simulink model "Wall_Model_Version_Final_2018a"  (R2018a)
settings: Solver=ode3  StartTime=0.0  StopTime=87000  FixedStep=Ts  RelTol=1e-3  EnableMultiTasking=on
InitFcn:
  | clc;
  | clear all;
  | close all;
  | addpath('D:\Aravind_A0164966M_EE5003\Matlab files\3r2c model')
  | Ts=1
  | Duration=36000;
  | %% Coefficients of Rs and Cs
  | 
  | %% Front Wall
  | l1 = 7.37;
  | b1 = 2.63;
  | y1 = 0.186;
  | x1 = 0.111;
  | y2 = 0.814;
  | x2 = 0.506;
  | x3 = 0.383;
  | 
  | %% Left Wall
  | l2 = 10.11;
  | b2 = 2.63;
  | y3 = 0.186;
  | x4 = 0.111;
  | y4 = 0.814;
  | x5 = 0.506;
  | x6 = 0.383;
  | 
  | %% Left Wall Glass
  | x4_g = 0.5;
  | x5_g = 0.5;
  | y3_g = 1;
  | 
  | %% Right Wall
  | l3 = 7.37;
  | b3 = 2.63;
  | y5 = 0.186;
  | x7 = 0.111;
  | y6 = 0.814;
  | x8 = 0.506;
  | x9 = 0.383;
  | 
  | %% Back Wall
  | l4 = 10.11;
  | b4 = 2.63;
  | y7 = 1;
  | x10 = 0.5;
  | %y8 = 0.5;
  | x11 = 0.5;
  | %x12= 0.33;
  | 
  | %% Roof
  | l5 = 10.11;
  | b5 = 7.37;
  | y9 = 0.186;
  | x13 = 0.111;
  | y10 = 0.814;
  | x14 = 0.506;
  | x15 = 0.383;
  | 
  | %% Floor
  | l6 = 10.11;
  | b6 = 7.37;
  | y11 = 0.186;
  | x16 = 0.111;
  | y12 = 0.814;
  | x17 = 0.506;
  | x18 = 0.383;
  | 
  | %%Areas
  | A1 = l1 * b1;
  | A2 = l2 * b2;
  | A3 = l3 * b3;
  | A4 = l4 * b4;
  | A5 = l5 * b5;
  | A6 = l6 * b6;
  | 
  | %% Initial Temperatures at the surfaces
  | T1_initial_front=301;
  | T2_initial_front=300;
  | 
  | T1_initial_left=301;
  | T2_initial_left=300;
  | 
  | T1_initial_right=301;
  | T2_initial_right=300;
  | 
  | T1_initial_back=301;
  | T2_initial_back=300;
  | 
  | T1_initial_roof=301;
  | T2_initial_roof=300;
  | 
  | T1_initial_floor=301;
  | T2_initial_floor=300;
  | 
  | %ri = 0.1300; % m2 K/W resistance of inner surface of brick wall
  | %rso = 0.04; % m2 K/W resistance of outer surface of the wall
  | 
  | ri = 0;
  | rso = 0;
  | %% Density of Building materials in the room
  | p_conc    = 2400; % kg/m3 density of concrete
  | p_pstr     = 850; % kg/m3 density of plastering
  | p_gb       = 1100; % kg/m3 density of gypsum board
  | p_glass    = 2530; % kg/m3 density of glass
  | p_swood  = 550;   % kg/m3 density of soft-wood
  | 
  | %% Thermal heat capacity of the building materials in the room
  | c_conc    = 840;  % J/kg K heat capacity of concrete
  | c_pstr     = 1000;  %J/kg K heat capacity of plastering
  | c_gb       = 700; % J/kg K heat capacity of gypsum board
  | c_glass    = 840;  % J/kg K heat capacity of glass
  | c_swood  = 1700; % J/kg K heat capacity of soft-wood
  | 
  | %% Thermal conductivity(lamda) of building materials in the room
  | l_conc    = 0.8;  % W/m K Thermal conductivity of concrete
  | l_pstr     = 0.013;  % W/m K Thermal conductivity of plastering
  | l_gb       = 0.35; % W/m K Thermal conductivity of gypsum board
  | l_glass    = 0.8;  % W/m K Thermal conductivity of glass
  | l_swood  = 0.08; % W/m K Thermal conductivity of soft-wood
  | 
  | %% Standard thickness of materials used
  | d_conc = 0.01;  % m Thickness of concrete BCA standard
  | d_pstr = 0.005; % m Thickness of plastering BCA standard
  | d_glass = 0.015; % m Thickness of glass wall widely used
  | d_swood = 0.01; % m Thickness of softwood on the right wall
  | d_gb = 0.015; % m Thickness of gypsum board
  | 
  | %% Resistance and Capacitance of front Wall
  | Rth1 =( ri + rso + (d_conc/l_conc) + (d_pstr/l_pstr))/(A1); % Thermal resistance
  | Cth1 = A1*(d_conc*p_conc*c_conc + d_pstr*p_pstr*c_pstr) ; % Thermal Capacitance
  | 
  | %% Resistance and Capacitance of left Wall concrete
  | A_conc = A2 * 0.5; % Half of the wall on the left is  glass wall
  | Rth2 =( ri + rso + (d_conc/l_conc) + (d_pstr/l_pstr))/(A_conc); % Thermal resistance
  | Cth2 = A_conc*(d_conc*p_conc*c_conc + d_pstr*p_pstr*c_pstr); % Thermal Capacitance
  | 
  | %% Resistance and Capacitance of left Wall glass
  | A_glass = A2 * 0.5; % Half of the wall on the left is  glass wall
  | Rth2_g =(d_glass/l_glass) /(A_glass); % Thermal resistance
  | Cth2_g = A_glass*(d_glass*p_glass*c_glass ); % Thermal Capacitance
  | 
  | %% Resistance and Capacitance of right Wall
  | Rth3 = ( ri + rso+ (d_conc/l_conc) + (d_swood/l_swood))/(A3);% Thermal resistance
  | Cth3 = A3*(d_swood*p_swood*c_swood + d_conc*p_conc*c_conc ); % Thermal Capacitance
  | 
  | %% Resistance and Capacitance of back Wall
  | Rth4 =(d_glass/l_glass) /(A4); % Thermal resistance
  | Cth4 = A4*(d_glass*p_glass*c_glass ); % Thermal Capacitance
  | 
  | %% Resistance and Capacitance of roof Wall
  | Rth5 = (d_gb/l_gb)/(A5);% Thermal resistance
  | Cth5 = A5*(d_gb*p_gb*c_gb ); % Thermal Capacitance
  | 
  | %% Resistance and Capacitance of floor Wall
  | Rth6 = (d_gb/l_gb)/(A6);% Thermal resistance
  | Cth6 = A6*(d_gb*p_gb*c_gb ); % Thermal Capacitance
  | 
  | %% Volume and mass of room
  | density_of_air = 1.184; % kg/m3 at 25 deg. K
  | volume = l1*l2*b1; % m3
  | mass = volume * density_of_air ;% kg
  | specific_heat = 1.005; % J/kg deg.K
  | tic;
  | 
  | Tleft = 298;
libraries: powerlib x72, simulink x1
(part 1 of 2)
settings Model: EnablePacing=on  Creator=elekkr  LastModifiedBy=accma
settings DataIOCC: LimitDataPoints=on  SaveFormat=Array
settings OptimizationCC: LifeSpan=inf
settings DebuggingCC: UnconnectedInputMsg=none  UnconnectedOutputMsg=none  UnconnectedLineMsg=none  SFUnexpectedBacktrackingDiag=warning  SFNoUnconditionalDefaultTransitionDiag=warning  SFExecutionAtInitializationDiag=none
settings HardwareCC: ProdBitPerPointer=32  ProdBitPerSizeT=32  ProdBitPerPtrDiffT=32  ProdLargestAtomicFloat=None  ProdIntDivRoundTo=Undefined  ProdEndianess=Unspecified  ProdWordSize=32  ProdHWDeviceType=32-bit Generic
settings ModelReferenceCC: PropagateSignalLabelsOutOfModel=off
settings CodeAppCC: StateflowObjectComments=on
settings GRTTargetCC: TargetLangStandard=C89/C90 (ANSI)  GeneratePreprocessorConditionals=Disable all
settings ConfigComp: CovMetricSettings=dw  CovHtmlReporting=on  CovSaveCumulativeToWorkspaceVar=on  CovSaveSingleToWorkspaceVar=on  CovExternalEMLEnable=off
settings SimscapeCC: SimscapeNormalizeSystem=off

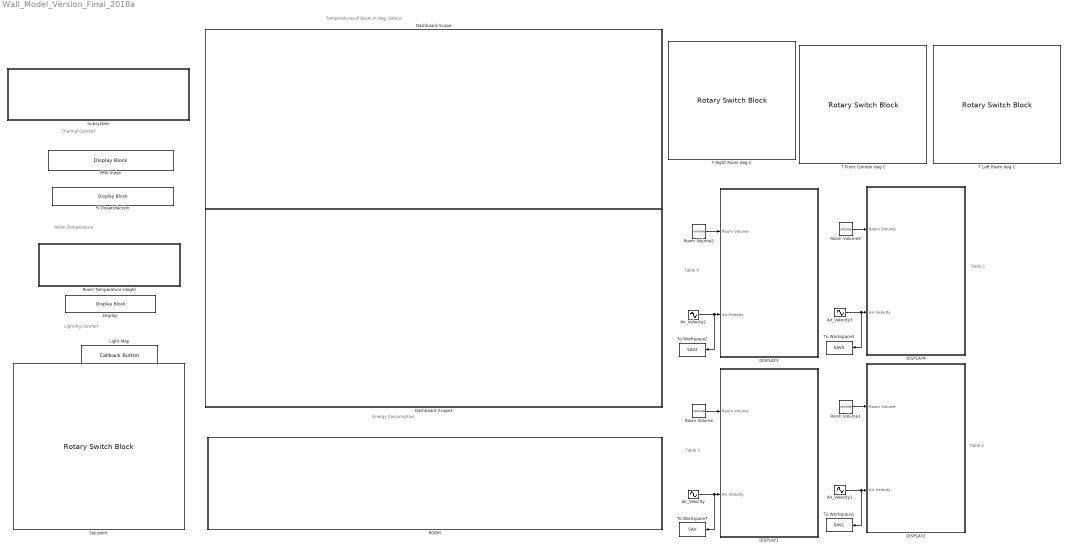
== system Wall_Model_Version_Final_2018a ==
  note: Table 1
  note: Thermal Comfort
  note: Lighting Comfort
  note: Temperatures of Room in deg. Celsius
  note: Energy Consumption
  note: Table 2
  note: Table 3
  note: Table 4
  note: Room Temperature
  % Dissatisfaction : DisplayBlock  WebBlockId=889  LabelPosition=Hide
  Air_Velocity{,1..3} (4 alike) : Sin  Amplitude=0.2  Bias=0.8  Frequency=2*pi/(12*3600)  SampleTime=0
  DISPLAY1 : Subsystem  mask(Sensor_node){}
      mask Display: fprintf('CO2 488.60 ppm\n\nCO 0.10 ppm\n\nHCHO 0.00 ppm\n\nO3 0.09 ppm\n\nPM2_5 0.03 ppm\n\nPM10 0.06 ppm\n\nAir Quality Index 14.82\n\n')
  DISPLAY2 : Subsystem  mask(Sensor_node){}
      mask Display: fprintf('CO2 491.84 ppm\n\nCO 0.11 ppm\n\nHCHO 0.00 ppm\n\nO3 0.08 ppm\n\nPM2_5 0.02 ppm\n\nPM10 0.02 ppm\n\nAir Quality Index 15.36\n\n')
  DISPLAY3 : Subsystem  mask(Sensor_node){}
      mask Display: fprintf('CO2 489.68 ppm\n\nCO 0.11 ppm\n\nHCHO 0.00 ppm\n\nO3 0.05 ppm\n\nPM2_5 0.05 ppm\n\nPM10 0.05 ppm\n\nAir Quality Index 15.00\n\n')
  DISPLAY4 : Subsystem  mask(Sensor_node){}
      mask Display: fprintf('CO2 489.68 ppm\n\nCO 0.09 ppm\n\nHCHO 0.00 ppm\n\nO3 0.08 ppm\n\nPM2_5 0.05 ppm\n\nPM10 0.04 ppm\n\nAir Quality Index 15.00\n\n')
  Dashboard Scope : Subsystem  DialogController=hmiCreateDDGDialog  IsWebBlock=on  mask(MWDashboardBlock){webBlockId=52df8120-a1fd-461c-886b-445e676d82b8, webBlockType=sdiscope, ShowInLibBrowser=on, ShowInitialText=on, HMISrcModelName=Wall_Model_Version_Final_2018a}
      mask prompts: webBlockId "WebBlock Id"; webBlockType "WebBlock Type"; HMISrcModelName "Source Model"
      mask help: Traces signals on the dashboard scope during simulation.
      mask Help: helpview([docroot '/mapfiles/simulink.map'], 'hmi_scope')
      mask Display:
      | if strcmp(get_param(bdroot(gcb),'BlockDiagramType'),'library')
      |  image([(matlabroot) '/toolbox/simulink/hmi/icons/SDIScope.png'])
      | end
  Dashboard Scope1 : Subsystem  DialogController=hmiCreateDDGDialog  IsWebBlock=on  mask(MWDashboardBlock){webBlockId=c0c79143-6636-452e-a0ed-83ee40a087d1, webBlockType=sdiscope, ShowInLibBrowser=on, ShowInitialText=on, HMISrcModelName=Wall_Model_Version_Final_2018a}
      mask prompts: webBlockId "WebBlock Id"; webBlockType "WebBlock Type"; HMISrcModelName "Source Model"
      mask help: Traces signals on the dashboard scope during simulation.
      mask Help: helpview([docroot '/mapfiles/simulink.map'], 'hmi_scope')
      mask Display:
      | if strcmp(get_param(bdroot(gcb),'BlockDiagramType'),'library')
      |  image([(matlabroot) '/toolbox/simulink/hmi/icons/SDIScope.png'])
      | end
  Display : DisplayBlock  WebBlockId=772  LabelPosition=Hide
  Light Map : CallbackButton  WebBlockId=904
      settings: ClickFcn=heatmap_V2
  PMV Index : DisplayBlock  WebBlockId=888  LabelPosition=Hide
  ROOM : Subsystem
  Room Temperature (degK) : Subsystem  DialogController=hmiCreateDDGDialog  IsWebBlock=on  mask(MWDashboardBlock){webBlockId=d421009d-199f-4938-a325-427fcb2645d5, webBlockType=lineargauge, ShowInLibBrowser=on, ShowInitialText=on, HMISrcModelName=Wall_Model_Version_Final_2018a}
      mask prompts: webBlockId "WebBlock Id"; webBlockType "WebBlock Type"; HMISrcModelName "Source Model"
      mask help: Display an input value on a linear scale.
      mask Help: helpview([docroot '/mapfiles/simulink.map'], 'hmi_linear_gauge')
      mask Display:
      | if strcmp(get_param(bdroot(gcb),'BlockDiagramType'),'library')
      |  image([(matlabroot) '/toolbox/simulink/hmi/icons/LinearGauge.png'])
      | end
  Room Volume{,1..3} (4 alike) : Constant  Value=volume
  Set-point : RotarySwitchBlock  WebBlockId=542  LabelPosition=Hide
      settings: Values={{'Cold', '', '', 'Optimum', '', '', '', '', '', '', 'Hot'}, [293 294 295 296 297 298 299 300 301 302 303]}
  Subsystem : Subsystem  mask(GBIC_Simulation time){}
      settings: AttributesFormatString=58.23
      mask Display: fprintf('Simulation_Time_Elapsed=28.00 seconds\nPhysical_Time_Elapsed=58.23 seconds\nSimulation_Speed=0.48 times')
  T Front Corridor deg.C : RotarySwitchBlock  WebBlockId=766  LabelPosition=Hide
      settings: Values={{'20', '21', '22', '23', '24', '25', '26', '27', '28', '29', '30', '31', '32'}, [293 294 295 296 297 298 299 300 301 302 303 304 305]}
  T Left Room deg.C : RotarySwitchBlock  WebBlockId=768  LabelPosition=Hide
      settings: Values={{'20', '21', '22', '23', '24', '25', '26', '27', '28', '29', '30', '31', '32'}, [293 294 295 296 297 298 299 300 301 302 303 304 305]}
  T Right Room deg.C : RotarySwitchBlock  WebBlockId=769  LabelPosition=Hide
      settings: Values={{'20', '21', '22', '23', '24', '25', '26', '27', '28', '29', '30', '31', '32'}, [293 294 295 296 297 298 299 300 301 302 303 304 305]}
  To Workspace1 : ToWorkspace  VariableName=SAV1  SaveFormat=Timeseries  SampleTime=-1
  To Workspace2 : ToWorkspace  VariableName=SAV2  SaveFormat=Timeseries  SampleTime=-1
  To Workspace3 : ToWorkspace  VariableName=SAV3  SaveFormat=Timeseries  SampleTime=-1
  To Workspace7 : ToWorkspace  VariableName=SAV  SaveFormat=Timeseries  SampleTime=-1
  wires:
  Room Volume/1 -> DISPLAY1/1(Room Volume)
  Air_Velocity/1 -> To Workspace7/1, DISPLAY1/2(Air Velocity)
  Air_Velocity1/1 -> To Workspace1/1, DISPLAY2/2(Air Velocity)
  Room Volume1/1 -> DISPLAY2/1(Room Volume)
  Air_Velocity2/1 -> To Workspace2/1, DISPLAY3/2(Air Velocity)
  Room Volume2/1 -> DISPLAY3/1(Room Volume)
  Room Volume3/1 -> DISPLAY4/1(Room Volume)
  Air_Velocity3/1 -> To Workspace3/1, DISPLAY4/2(Air Velocity)

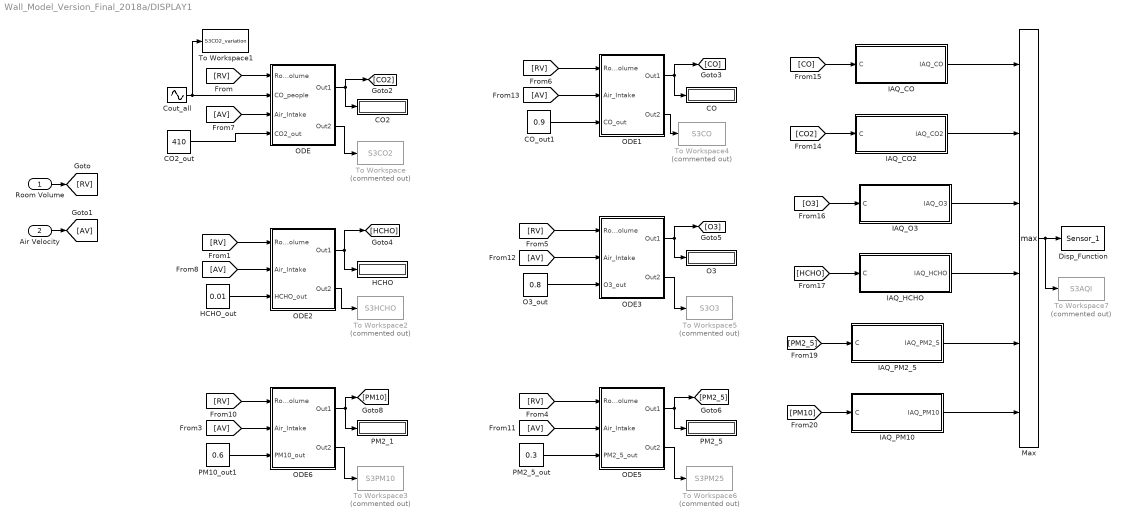
== system Wall_Model_Version_Final_2018a/DISPLAY1 ==
  Room Volume : Inport
  Air Velocity : Inport  Port=2
  CO : Display
  CO2 : Display
  CO2_out : Constant  Value=410
  CO_out1 : Constant  Value=0.9
  Cout_all : Sin  Amplitude=50  Bias=450  Frequency=2*pi/(24*3600)  SampleTime=0
  Disp_Function : M-S-Function  FunctionName=Sensor_1
  HCHO : Display
  HCHO_out : Constant  Value=0.01
  IAQ_CO : MATLAB Function  TreatAsAtomicUnit=on
  IAQ_CO2 : MATLAB Function  TreatAsAtomicUnit=on
  IAQ_HCHO : MATLAB Function  TreatAsAtomicUnit=on
  IAQ_O3 : MATLAB Function  TreatAsAtomicUnit=on
  IAQ_PM10 : MATLAB Function  TreatAsAtomicUnit=on
  IAQ_PM2_5 : MATLAB Function  TreatAsAtomicUnit=on
  Max : MinMax  Function=max  Inputs=6
  O3 : Display
  O3_out : Constant  Value=0.8
  ODE : Subsystem
  ODE1 : Subsystem
  ODE2 : Subsystem
  ODE3 : Subsystem
  ODE5 : Subsystem
  ODE6 : Subsystem
  PM10_out1 : Constant  Value=0.6
  PM2_1 : Display
  PM2_5 : Display
  PM2_5_out : Constant  Value=0.3
  To Workspace : ToWorkspace  Commented=on  VariableName=S3CO2  SaveFormat=Timeseries  SampleTime=-1
  To Workspace1 : ToWorkspace  VariableName=S3CO2_variation  SaveFormat=Timeseries  SampleTime=-1
  To Workspace2 : ToWorkspace  Commented=on  VariableName=S3HCHO  SaveFormat=Timeseries  SampleTime=-1
  To Workspace3 : ToWorkspace  Commented=on  VariableName=S3PM10  SaveFormat=Timeseries  SampleTime=-1
  To Workspace4 : ToWorkspace  Commented=on  VariableName=S3CO  SaveFormat=Timeseries  SampleTime=-1
  To Workspace5 : ToWorkspace  Commented=on  VariableName=S3O3  SaveFormat=Timeseries  SampleTime=-1
  To Workspace6 : ToWorkspace  Commented=on  VariableName=S3PM25  SaveFormat=Timeseries  SampleTime=-1
  To Workspace7 : ToWorkspace  Commented=on  VariableName=S3AQI  SaveFormat=Timeseries  SampleTime=-1
  wires:
  Cout_all/1 -> To Workspace1/1, ODE/2(CO_people)
  ODE2/1(Out1) -> HCHO/1, [HCHO]
  HCHO_out/1 -> ODE2/3(HCHO_out)
  CO_out1/1 -> ODE1/3(CO_out)
  CO2_out/1 -> ODE/4(CO2_out)
  O3_out/1 -> ODE3/3(O3_out)
  ODE3/1(Out1) -> O3/1, [O3]
  IAQ_CO/1(IAQ_CO) -> Max/1
  IAQ_HCHO/1(IAQ_HCHO) -> Max/4
  ODE/1(Out1) -> CO2/1, [CO2]
  IAQ_CO2/1(IAQ_CO2) -> Max/2
  ODE1/1(Out1) -> CO/1, [CO]
  IAQ_O3/1(IAQ_O3) -> Max/3
  ODE5/1(Out1) -> PM2_5/1, [PM2_5]
  PM2_5_out/1 -> ODE5/3(PM2_5_out)
  [RV] -> ODE/1(Room_Volume)
  [RV] -> ODE2/1(Room_Volume)
  [RV] -> ODE5/1(Room_Volume)
  [RV] -> ODE3/1(Room_Volume)
  [RV] -> ODE1/1(Room_Volume)
  [AV] -> ODE/3(Air_Intake)
  [AV] -> ODE2/2(Air_Intake)
  [AV] -> ODE5/2(Air_Intake)
  [AV] -> ODE3/2(Air_Intake)
  [AV] -> ODE1/2(Air_Intake)
  [AV] -> ODE6/2(Air_Intake)
  [RV] -> ODE6/1(Room_Volume)
  PM10_out1/1 -> ODE6/3(PM10_out)
  [CO2] -> IAQ_CO2/1(C)
  [CO] -> IAQ_CO/1(C)
  [O3] -> IAQ_O3/1(C)
  [HCHO] -> IAQ_HCHO/1(C)
  [PM2_5] -> IAQ_PM2_5/1(C)
  [PM10] -> IAQ_PM10/1(C)
  ODE6/1(Out1) -> PM2_1/1, [PM10]
  Max/1 -> To Workspace7/1, Disp_Function/1
  IAQ_PM2_5/1(IAQ_PM2_5) -> Max/5
  IAQ_PM10/1(IAQ_PM10) -> Max/6
  Room Volume/1 -> [RV]
  Air Velocity/1 -> [AV]
  ODE/2(Out2) -> To Workspace/1
  ODE2/2(Out2) -> To Workspace2/1
  ODE6/2(Out2) -> To Workspace3/1
  ODE1/2(Out2) -> To Workspace4/1
  ODE3/2(Out2) -> To Workspace5/1
  ODE5/2(Out2) -> To Workspace6/1

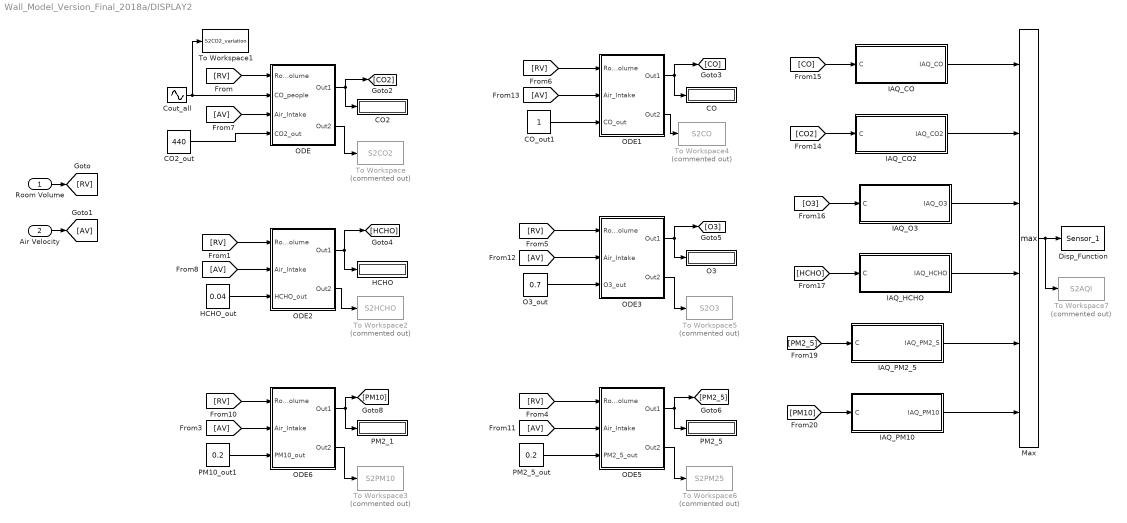
== system Wall_Model_Version_Final_2018a/DISPLAY2 ==
  Room Volume : Inport
  Air Velocity : Inport  Port=2
  CO : Display
  CO2 : Display
  CO2_out : Constant  Value=440
  CO_out1 : Constant
  Cout_all : Sin  Amplitude=50  Bias=450  Frequency=2*pi/(24*3600)  SampleTime=0
  Disp_Function : M-S-Function  FunctionName=Sensor_1
  HCHO : Display
  HCHO_out : Constant  Value=0.04
  IAQ_CO : MATLAB Function  TreatAsAtomicUnit=on
  IAQ_CO2 : MATLAB Function  TreatAsAtomicUnit=on
  IAQ_HCHO : MATLAB Function  TreatAsAtomicUnit=on
  IAQ_O3 : MATLAB Function  TreatAsAtomicUnit=on
  IAQ_PM10 : MATLAB Function  TreatAsAtomicUnit=on
  IAQ_PM2_5 : MATLAB Function  TreatAsAtomicUnit=on
  Max : MinMax  Function=max  Inputs=6
  O3 : Display
  O3_out : Constant  Value=0.7
  ODE : Subsystem
  ODE1 : Subsystem
  ODE2 : Subsystem
  ODE3 : Subsystem
  ODE5 : Subsystem
  ODE6 : Subsystem
  PM10_out1 : Constant  Value=0.2
  PM2_1 : Display
  PM2_5 : Display
  PM2_5_out : Constant  Value=0.2
  To Workspace : ToWorkspace  Commented=on  VariableName=S2CO2  SaveFormat=Timeseries  SampleTime=-1
  To Workspace1 : ToWorkspace  VariableName=S2CO2_variation  SaveFormat=Timeseries  SampleTime=-1
  To Workspace2 : ToWorkspace  Commented=on  VariableName=S2HCHO  SaveFormat=Timeseries  SampleTime=-1
  To Workspace3 : ToWorkspace  Commented=on  VariableName=S2PM10  SaveFormat=Timeseries  SampleTime=-1
  To Workspace4 : ToWorkspace  Commented=on  VariableName=S2CO  SaveFormat=Timeseries  SampleTime=-1
  To Workspace5 : ToWorkspace  Commented=on  VariableName=S2O3  SaveFormat=Timeseries  SampleTime=-1
  To Workspace6 : ToWorkspace  Commented=on  VariableName=S2PM25  SaveFormat=Timeseries  SampleTime=-1
  To Workspace7 : ToWorkspace  Commented=on  VariableName=S2AQI  SaveFormat=Timeseries  SampleTime=-1
  wires:
  Cout_all/1 -> To Workspace1/1, ODE/2(CO_people)
  ODE2/1(Out1) -> HCHO/1, [HCHO]
  HCHO_out/1 -> ODE2/3(HCHO_out)
  CO_out1/1 -> ODE1/3(CO_out)
  CO2_out/1 -> ODE/4(CO2_out)
  O3_out/1 -> ODE3/3(O3_out)
  ODE3/1(Out1) -> O3/1, [O3]
  IAQ_CO/1(IAQ_CO) -> Max/1
  IAQ_HCHO/1(IAQ_HCHO) -> Max/4
  ODE/1(Out1) -> CO2/1, [CO2]
  IAQ_CO2/1(IAQ_CO2) -> Max/2
  ODE1/1(Out1) -> CO/1, [CO]
  IAQ_O3/1(IAQ_O3) -> Max/3
  ODE5/1(Out1) -> PM2_5/1, [PM2_5]
  PM2_5_out/1 -> ODE5/3(PM2_5_out)
  [RV] -> ODE/1(Room_Volume)
  [RV] -> ODE2/1(Room_Volume)
  [RV] -> ODE5/1(Room_Volume)
  [RV] -> ODE3/1(Room_Volume)
  [RV] -> ODE1/1(Room_Volume)
  [AV] -> ODE/3(Air_Intake)
  [AV] -> ODE2/2(Air_Intake)
  [AV] -> ODE5/2(Air_Intake)
  [AV] -> ODE3/2(Air_Intake)
  [AV] -> ODE1/2(Air_Intake)
  [AV] -> ODE6/2(Air_Intake)
  [RV] -> ODE6/1(Room_Volume)
  PM10_out1/1 -> ODE6/3(PM10_out)
  [CO2] -> IAQ_CO2/1(C)
  [CO] -> IAQ_CO/1(C)
  [O3] -> IAQ_O3/1(C)
  [HCHO] -> IAQ_HCHO/1(C)
  [PM2_5] -> IAQ_PM2_5/1(C)
  [PM10] -> IAQ_PM10/1(C)
  ODE6/1(Out1) -> PM2_1/1, [PM10]
  Max/1 -> To Workspace7/1, Disp_Function/1
  IAQ_PM2_5/1(IAQ_PM2_5) -> Max/5
  IAQ_PM10/1(IAQ_PM10) -> Max/6
  Room Volume/1 -> [RV]
  Air Velocity/1 -> [AV]
  ODE/2(Out2) -> To Workspace/1
  ODE2/2(Out2) -> To Workspace2/1
  ODE6/2(Out2) -> To Workspace3/1
  ODE1/2(Out2) -> To Workspace4/1
  ODE3/2(Out2) -> To Workspace5/1
  ODE5/2(Out2) -> To Workspace6/1

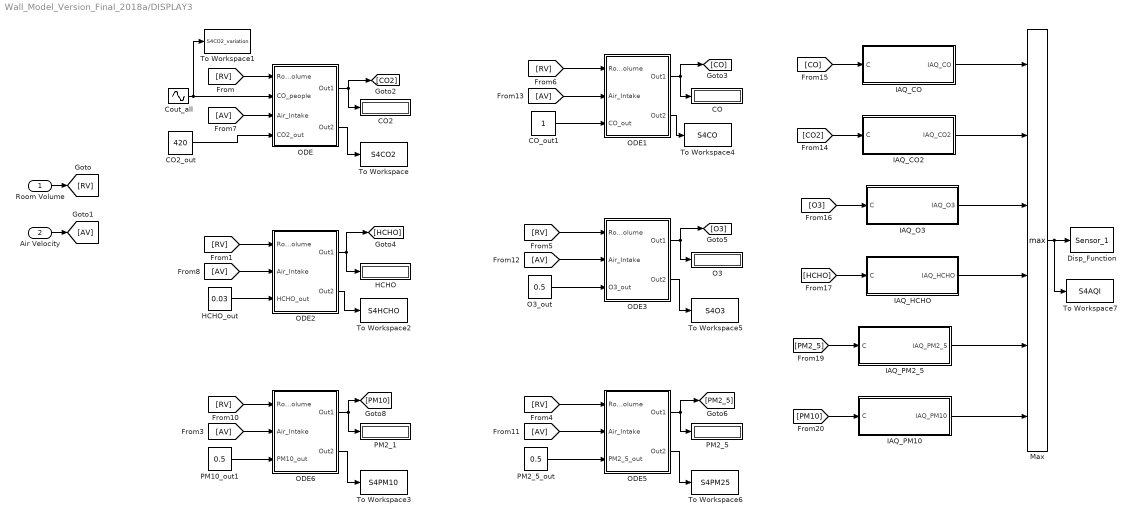
== system Wall_Model_Version_Final_2018a/DISPLAY3 ==
  Room Volume : Inport
  Air Velocity : Inport  Port=2
  CO : Display
  CO2 : Display
  CO2_out : Constant  Value=420
  CO_out1 : Constant
  Cout_all : Sin  Amplitude=50  Bias=450  Frequency=2*pi/(24*3600)  SampleTime=0
  Disp_Function : M-S-Function  FunctionName=Sensor_1
  HCHO : Display
  HCHO_out : Constant  Value=0.03
  IAQ_CO : MATLAB Function  TreatAsAtomicUnit=on
  IAQ_CO2 : MATLAB Function  TreatAsAtomicUnit=on
  IAQ_HCHO : MATLAB Function  TreatAsAtomicUnit=on
  IAQ_O3 : MATLAB Function  TreatAsAtomicUnit=on
  IAQ_PM10 : MATLAB Function  TreatAsAtomicUnit=on
  IAQ_PM2_5 : MATLAB Function  TreatAsAtomicUnit=on
  Max : MinMax  Function=max  Inputs=6
  O3 : Display
  O3_out : Constant  Value=0.5
  ODE : Subsystem
  ODE1 : Subsystem
  ODE2 : Subsystem
  ODE3 : Subsystem
  ODE5 : Subsystem
  ODE6 : Subsystem
  PM10_out1 : Constant  Value=0.5
  PM2_1 : Display
  PM2_5 : Display
  PM2_5_out : Constant  Value=0.5
  To Workspace : ToWorkspace  VariableName=S4CO2  SaveFormat=Timeseries  SampleTime=-1
  To Workspace1 : ToWorkspace  VariableName=S4CO2_variation  SaveFormat=Timeseries  SampleTime=-1
  To Workspace2 : ToWorkspace  VariableName=S4HCHO  SaveFormat=Timeseries  SampleTime=-1
  To Workspace3 : ToWorkspace  VariableName=S4PM10  SaveFormat=Timeseries  SampleTime=-1
  To Workspace4 : ToWorkspace  VariableName=S4CO  SaveFormat=Timeseries  SampleTime=-1
  To Workspace5 : ToWorkspace  VariableName=S4O3  SaveFormat=Timeseries  SampleTime=-1
  To Workspace6 : ToWorkspace  VariableName=S4PM25  SaveFormat=Timeseries  SampleTime=-1
  To Workspace7 : ToWorkspace  VariableName=S4AQI  SaveFormat=Timeseries  SampleTime=-1
  wires:
  Cout_all/1 -> To Workspace1/1, ODE/2(CO_people)
  ODE2/1(Out1) -> HCHO/1, [HCHO]
  HCHO_out/1 -> ODE2/3(HCHO_out)
  CO_out1/1 -> ODE1/3(CO_out)
  CO2_out/1 -> ODE/4(CO2_out)
  O3_out/1 -> ODE3/3(O3_out)
  ODE3/1(Out1) -> O3/1, [O3]
  IAQ_CO/1(IAQ_CO) -> Max/1
  IAQ_HCHO/1(IAQ_HCHO) -> Max/4
  ODE/1(Out1) -> CO2/1, [CO2]
  IAQ_CO2/1(IAQ_CO2) -> Max/2
  ODE1/1(Out1) -> CO/1, [CO]
  IAQ_O3/1(IAQ_O3) -> Max/3
  ODE5/1(Out1) -> PM2_5/1, [PM2_5]
  PM2_5_out/1 -> ODE5/3(PM2_5_out)
  [RV] -> ODE/1(Room_Volume)
  [RV] -> ODE2/1(Room_Volume)
  [RV] -> ODE5/1(Room_Volume)
  [RV] -> ODE3/1(Room_Volume)
  [RV] -> ODE1/1(Room_Volume)
  [AV] -> ODE/3(Air_Intake)
  [AV] -> ODE2/2(Air_Intake)
  [AV] -> ODE5/2(Air_Intake)
  [AV] -> ODE3/2(Air_Intake)
  [AV] -> ODE1/2(Air_Intake)
  [AV] -> ODE6/2(Air_Intake)
  [RV] -> ODE6/1(Room_Volume)
  PM10_out1/1 -> ODE6/3(PM10_out)
  [CO2] -> IAQ_CO2/1(C)
  [CO] -> IAQ_CO/1(C)
  [O3] -> IAQ_O3/1(C)
  [HCHO] -> IAQ_HCHO/1(C)
  [PM2_5] -> IAQ_PM2_5/1(C)
  [PM10] -> IAQ_PM10/1(C)
  ODE6/1(Out1) -> PM2_1/1, [PM10]
  Max/1 -> To Workspace7/1, Disp_Function/1
  IAQ_PM2_5/1(IAQ_PM2_5) -> Max/5
  IAQ_PM10/1(IAQ_PM10) -> Max/6
  Room Volume/1 -> [RV]
  Air Velocity/1 -> [AV]
  ODE/2(Out2) -> To Workspace/1
  ODE2/2(Out2) -> To Workspace2/1
  ODE6/2(Out2) -> To Workspace3/1
  ODE1/2(Out2) -> To Workspace4/1
  ODE3/2(Out2) -> To Workspace5/1
  ODE5/2(Out2) -> To Workspace6/1

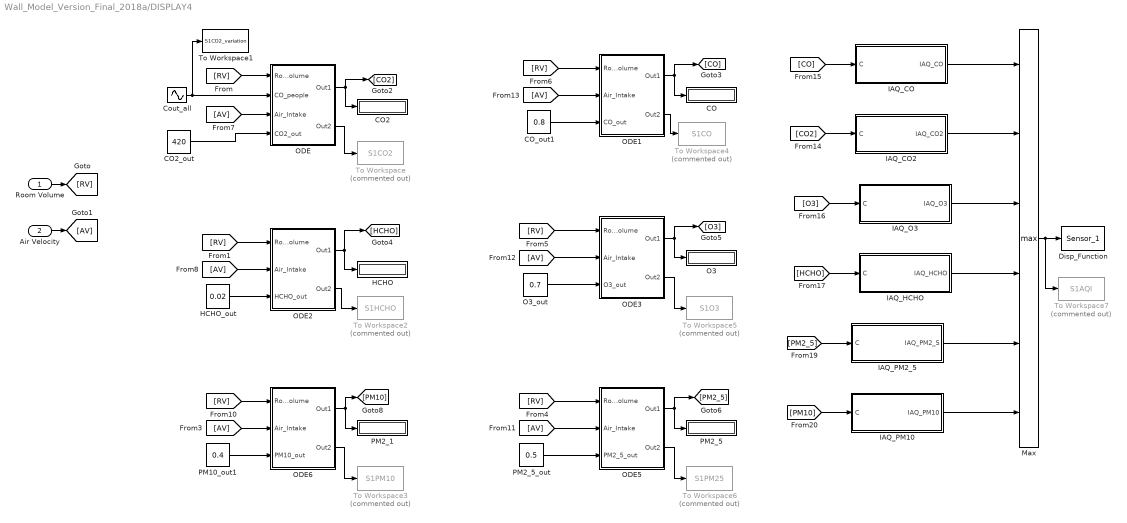
== system Wall_Model_Version_Final_2018a/DISPLAY4 ==
  Room Volume : Inport
  Air Velocity : Inport  Port=2
  CO : Display
  CO2 : Display
  CO2_out : Constant  Value=420
  CO_out1 : Constant  Value=0.8
  Cout_all : Sin  Amplitude=50  Bias=450  Frequency=2*pi/(24*3600)  SampleTime=0
  Disp_Function : M-S-Function  FunctionName=Sensor_1
  HCHO : Display
  HCHO_out : Constant  Value=0.02
  IAQ_CO : MATLAB Function  TreatAsAtomicUnit=on
  IAQ_CO2 : MATLAB Function  TreatAsAtomicUnit=on
  IAQ_HCHO : MATLAB Function  TreatAsAtomicUnit=on
  IAQ_O3 : MATLAB Function  TreatAsAtomicUnit=on
  IAQ_PM10 : MATLAB Function  TreatAsAtomicUnit=on
  IAQ_PM2_5 : MATLAB Function  TreatAsAtomicUnit=on
  Max : MinMax  Function=max  Inputs=6
  O3 : Display
  O3_out : Constant  Value=0.7
  ODE : Subsystem
  ODE1 : Subsystem
  ODE2 : Subsystem
  ODE3 : Subsystem
  ODE5 : Subsystem
  ODE6 : Subsystem
  PM10_out1 : Constant  Value=0.4
  PM2_1 : Display
  PM2_5 : Display
  PM2_5_out : Constant  Value=0.5
  To Workspace : ToWorkspace  Commented=on  VariableName=S1CO2  SaveFormat=Timeseries  SampleTime=-1
  To Workspace1 : ToWorkspace  VariableName=S1CO2_variation  SaveFormat=Timeseries  SampleTime=-1
  To Workspace2 : ToWorkspace  Commented=on  VariableName=S1HCHO  SaveFormat=Timeseries  SampleTime=-1
  To Workspace3 : ToWorkspace  Commented=on  VariableName=S1PM10  SaveFormat=Timeseries  SampleTime=-1
  To Workspace4 : ToWorkspace  Commented=on  VariableName=S1CO  SaveFormat=Timeseries  SampleTime=-1
  To Workspace5 : ToWorkspace  Commented=on  VariableName=S1O3  SaveFormat=Timeseries  SampleTime=-1
  To Workspace6 : ToWorkspace  Commented=on  VariableName=S1PM25  SaveFormat=Timeseries  SampleTime=-1
  To Workspace7 : ToWorkspace  Commented=on  VariableName=S1AQI  SaveFormat=Timeseries  SampleTime=-1
  wires:
  Cout_all/1 -> To Workspace1/1, ODE/2(CO_people)
  ODE2/1(Out1) -> HCHO/1, [HCHO]
  HCHO_out/1 -> ODE2/3(HCHO_out)
  CO_out1/1 -> ODE1/3(CO_out)
  CO2_out/1 -> ODE/4(CO2_out)
  O3_out/1 -> ODE3/3(O3_out)
  ODE3/1(Out1) -> O3/1, [O3]
  IAQ_CO/1(IAQ_CO) -> Max/1
  IAQ_HCHO/1(IAQ_HCHO) -> Max/4
  ODE/1(Out1) -> CO2/1, [CO2]
  IAQ_CO2/1(IAQ_CO2) -> Max/2
  ODE1/1(Out1) -> CO/1, [CO]
  IAQ_O3/1(IAQ_O3) -> Max/3
  ODE5/1(Out1) -> PM2_5/1, [PM2_5]
  PM2_5_out/1 -> ODE5/3(PM2_5_out)
  [RV] -> ODE/1(Room_Volume)
  [RV] -> ODE2/1(Room_Volume)
  [RV] -> ODE5/1(Room_Volume)
  [RV] -> ODE3/1(Room_Volume)
  [RV] -> ODE1/1(Room_Volume)
  [AV] -> ODE/3(Air_Intake)
  [AV] -> ODE2/2(Air_Intake)
  [AV] -> ODE5/2(Air_Intake)
  [AV] -> ODE3/2(Air_Intake)
  [AV] -> ODE1/2(Air_Intake)
  [AV] -> ODE6/2(Air_Intake)
  [RV] -> ODE6/1(Room_Volume)
  PM10_out1/1 -> ODE6/3(PM10_out)
  [CO2] -> IAQ_CO2/1(C)
  [CO] -> IAQ_CO/1(C)
  [O3] -> IAQ_O3/1(C)
  [HCHO] -> IAQ_HCHO/1(C)
  [PM2_5] -> IAQ_PM2_5/1(C)
  [PM10] -> IAQ_PM10/1(C)
  ODE6/1(Out1) -> PM2_1/1, [PM10]
  Max/1 -> To Workspace7/1, Disp_Function/1
  IAQ_PM2_5/1(IAQ_PM2_5) -> Max/5
  IAQ_PM10/1(IAQ_PM10) -> Max/6
  Room Volume/1 -> [RV]
  Air Velocity/1 -> [AV]
  ODE/2(Out2) -> To Workspace/1
  ODE2/2(Out2) -> To Workspace2/1
  ODE6/2(Out2) -> To Workspace3/1
  ODE1/2(Out2) -> To Workspace4/1
  ODE3/2(Out2) -> To Workspace5/1
  ODE5/2(Out2) -> To Workspace6/1

== system Wall_Model_Version_Final_2018a/Dashboard Scope ==

== system Wall_Model_Version_Final_2018a/Dashboard Scope1 ==

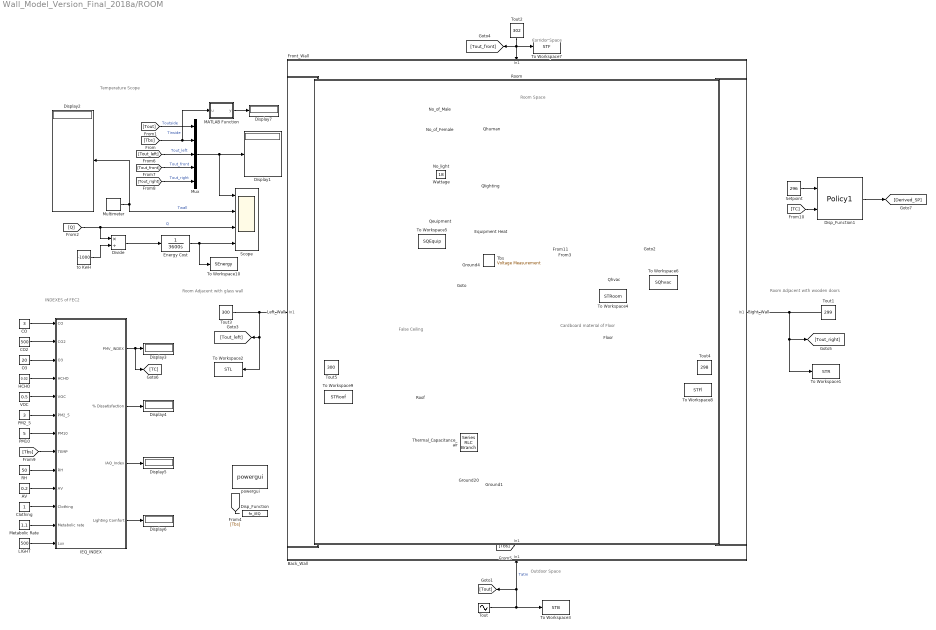
== system Wall_Model_Version_Final_2018a/ROOM ==
  note: False Ceiling
  note: Cardboard material of Floor
  note: Room Adjacent with wooden doors
  note: Corridor Space
  note: Room Adjacent with glass wall
  note: Outdoor Space
  note: Room Space
  note: Temperature Scope
  note: INDEXES of FEC2
  AV : Constant  Value=0.2
  Back_Wall : Subsystem
      mask Display: fprintf('Temperature Outside= 30.00 deg. C\n')
  CO : Constant  Value=3
  CO2 : Constant  Value=500
  Clothing : Constant
  Disp_Function : M-S-Function  FunctionName=fn_IEQ
  Disp_Function1 : M-S-Function  FunctionName=Policy1
  Display{1..7} (7 alike) : Display
  Divide : Product  Inputs=*/
  Energy Cost : TransferFcn  Denominator=[3600 0]
  Equipment Heat : Subsystem
  Floor : Subsystem
      mask Display: fprintf('Temperature \n Below= \n25.00 deg. C\n')
  Front_Wall : Subsystem
      mask Display: fprintf('Temperature Corridor= 29.00 deg. C\n')
  Ground1 : powerlib/Elements/Ground  LConnTagsString=a
      settings: SourceProductName=Simscape Electrical
  Ground20 : powerlib/Elements/Ground  LConnTagsString=a
      settings: SourceProductName=Simscape Electrical
  Ground4 : powerlib/Elements/Ground  LConnTagsString=a
      settings: SourceProductName=Simscape Electrical
  HCHO : Constant  Value=0.02
  IEQ_INDEX : Subsystem
  LIGHT : Constant  Value=500
  Left_Wall : Subsystem
      mask Display: fprintf('Temperature \n Left Room= \n27.00 deg. C\n')
  MATLAB Function : MATLAB Function  TreatAsAtomicUnit=on
  Metabolic Rate : Constant  Value=1.1
  Multimeter : powerlib/Measurements/Multimeter  PhasorSimulation=off  OutputType=Complex  sel=1  L=10  Gain=0  yselected={}  PSBOutputType=1  PSBequivalent=0  AxesSetting=[0,0.1,-100,100]  Display=0  SavedBlockNames=-11
      settings: SourceProductName=Simscape Electrical
  Mux : Mux  Inputs=5
  No_light : Constant  Value=60
  No_of_Female : Sin  Amplitude=4  Bias=4  Frequency=2*pi/(24*3600)
  No_of_Male : Sin  Amplitude=4  Bias=4  Frequency=2*pi/(24*3600)
  O3 : Constant  Value=20
  PM10 : Constant  Value=5
  PM2_5 : Constant  Value=3
  Qeuipment : Sin  Amplitude=200  Bias=3200  Frequency=2*pi/(24*3600)  SampleTime=0
  Qhuman : Subsystem
  Qhvac : Subsystem
  Qlighting : Subsystem
  RH : Constant  Value=50
  Right_Wall : Subsystem
      mask Display: fprintf('Temperature \n Right Room= \n26.00 deg. C\n')
  Roof : Subsystem
      mask Display: fprintf('Temperature \n Above Roof= \n27.00 deg. C\n')
  Room : Subsystem
      mask Display: fprintf('Temperature Room= 27.35 deg. C\n')
  Scope : Scope  NumInputPorts=4
  Setpoint : Constant  Value=296
  Tbs : powerlib/Measurements/Voltage Measurement  PhasorSimulation=off  OutputType=Magnitude  PSBequivalent=0
      settings: SourceProductName=Simscape Electrical
  Thermal_Capacitance_air : powerlib/Elements/Series RLC Branch  LConnTagsString=__new0  RConnTagsString=__new0  BranchType=C  Resistance=0  Inductance=1e-3  SetiL0=off  InitialCurrent=0  Capacitance=density_of_air * volume * specific_heat  Setx0=on  InitialVoltage=298  Measurements=Branch voltage
      settings: SourceProductName=Simscape Electrical
  To Workspace1 : ToWorkspace  VariableName=STR  SaveFormat=Timeseries  SampleTime=-1
  To Workspace10 : ToWorkspace  VariableName=SEnergy  SaveFormat=Timeseries  SampleTime=-1
  To Workspace2 : ToWorkspace  VariableName=STL  SaveFormat=Timeseries  SampleTime=-1
  To Workspace3 : ToWorkspace  VariableName=STB  SaveFormat=Timeseries  SampleTime=-1
  To Workspace4 : ToWorkspace  VariableName=STRoom  SaveFormat=Timeseries  SampleTime=-1
  To Workspace5 : ToWorkspace  VariableName=SQEquip  SaveFormat=Timeseries  SampleTime=-1
  To Workspace6 : ToWorkspace  VariableName=SQhvac  SaveFormat=Timeseries  SampleTime=-1
  To Workspace7 : ToWorkspace  VariableName=STF  SaveFormat=Timeseries  SampleTime=-1
  To Workspace8 : ToWorkspace  VariableName=STFl  SaveFormat=Timeseries  SampleTime=-1
  To Workspace9 : ToWorkspace  VariableName=STRoof  SaveFormat=Timeseries  SampleTime=-1
  Tout : Sin  Amplitude=1.5  Bias=303  Frequency=2*pi/(24*3600)  SampleTime=0
  Tout1 : Constant  Value=299
  Tout2 : Constant  Value=302
  Tout3 : Constant  Value=300
  Tout4 : Constant  Value=298
  Tout5 : Constant  Value=300
  VOC : Constant  Value=0.5
  Wattage : Constant  Value=18
  powergui : powerlib/powergui  Priority=1  SimulationMode=Discrete  SampleTime=Ts  frequency=60  Iterations=50  frequencyindice=0  Pbase=100e6  ErrMax=1e-4  UnitsV=kV  UnitsW=MW  buscounter=0  FunctionMessages=off  echomessages=off  EnableUseOfTLC=off  CurrentSourceSwitches=off  DisableSnubberDevices=off  DisableRonSwitches=off  DisableVfSwitches=off  DisplayEquations=off  SolverType=Tustin/Backward Euler (TBE)  Interpol=off  ExternalGateDelay=off  methode=off  Ts=100  x0status=blocks  SPID=off  SwTol=0  HookPort=off  RestoreLinks=warning  ResistiveCurrentMeasurement=off  Frange=[0:2:500]  Ylog=off  Xlog=on  ShowGrid=off  save=off  variable=ZData  structure=0  ZoomFFT=off  StartTime=0.0  cycles=1  DisplayStyle=1  fundamental=60  FreqAxis=off  MaxFrequency=1000  frequencyindicesteady=1  RmsSteady=1  display=off
  to KwH : Constant  Value=-1000
  wires:
  No_of_Female/1 -> Qhuman/2(No_Female)
  Tout5/1 -> To Workspace9/1, Roof/1(In1)
  Tout3/1 -> To Workspace2/1, [Tout_left], Left_Wall/1(In1)
  [Derived_SP] -> Qhvac/1(Setpoint)
  Qhvac/1(Qhvac) -> [Q]
  Tout/1 -> [Tout], Back_Wall/1(In1), To Workspace3/1  "Tatm"
  Tout4/1 -> To Workspace8/1, Floor/1(In1)
  No_light/1 -> Qlighting/1("No_light ")
  No_of_Male/1 -> Qhuman/1("No_Male ")
  Wattage/1 -> Qlighting/2(Wattage)
  Qeuipment/1 -> Equipment Heat/1(In1), To Workspace5/1
  Tbs/1 -> [Tbs]
  [Tbs] -> To Workspace4/1, Qhvac/2(Tbs)
  [Tbs] -> Room/1(In1)
  Tout1/1 -> To Workspace1/1, [Tout_right], Right_Wall/1(In1)
  Tout2/1 -> To Workspace7/1, [Tout_front], Front_Wall/1(In1)
  [Tbs] -> MATLAB Function/1(u), Mux/2  "Tinside"
  [Q] -> Scope/3, Divide/1  "Q"
  [Tout_right] -> Mux/5  "Tout_right"
  [Tout_front] -> Mux/4  "Tout_front"
  Multimeter/1 -> Scope/2, Display2/1  "Twall"
  Divide/1 -> Energy Cost/1
  to KwH/1 -> Divide/2
  Mux/1 -> Display1/1, Scope/1
  [Tout] -> Mux/1  "Toutside"
  Energy Cost/1 -> To Workspace10/1, Scope/4
  [Tout_left] -> Mux/3  "Tout_left"
  [Tbs] -> ?
  CO/1 -> IEQ_INDEX/1(CO)
  IEQ_INDEX/1(PMV_INDEX) -> [TC], Display3/1
  Clothing/1 -> IEQ_INDEX/11(Clothing)
  AV/1 -> IEQ_INDEX/10(AV)
  RH/1 -> IEQ_INDEX/9(RH)
  HCHO/1 -> IEQ_INDEX/4(HCHO)
  VOC/1 -> IEQ_INDEX/5(VOC)
  PM2_5/1 -> IEQ_INDEX/6(PM2_5)
  [Tbs] -> IEQ_INDEX/8(TEMP)
  Metabolic Rate/1 -> IEQ_INDEX/12(Metabolic rate)
  IEQ_INDEX/2("% Dissatisfaction ") -> Display4/1
  IEQ_INDEX/3(IAQ_Index) -> Display5/1
  PM10/1 -> IEQ_INDEX/7(PM10)
  CO2/1 -> IEQ_INDEX/2(CO2)
  LIGHT/1 -> IEQ_INDEX/13(Lux)
  O3/1 -> IEQ_INDEX/3(O3)
  IEQ_INDEX/4(Lighting Comfort) -> Display6/1
  Qhvac/2(Out2) -> To Workspace6/1
  Setpoint/1 -> Disp_Function1/1
  [TC] -> Disp_Function1/2
  Disp_Function1/1 -> [Derived_SP]
  MATLAB Function/1(y) -> Display7/1
  connections:
  Ground4/LConn1 -- Tbs/LConn2
  Equipment Heat/RConn1 -- Qhvac/RConn1 -- Right_Wall/RConn1 -- Back_Wall/RConn1 -- Roof/RConn1 -- Floor/RConn1 -- Left_Wall/RConn1 -- Tbs/LConn1 -- Qlighting/RConn1 -- Qhuman/RConn1 -- Front_Wall/RConn1
  Ground20/LConn1 -- Thermal_Capacitance_air/RConn1
  Thermal_Capacitance_air/LConn1 -- Ground1/LConn1

== system Wall_Model_Version_Final_2018a/Room Temperature (degK) ==

== system Wall_Model_Version_Final_2018a/Subsystem ==
  Disp_Function : M-S-Function  FunctionName=fn_Display

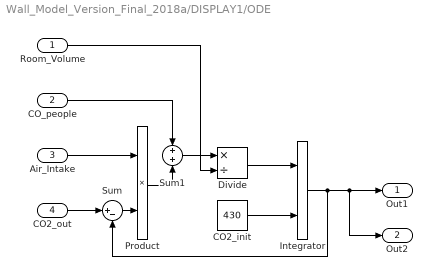
== system Wall_Model_Version_Final_2018a/DISPLAY1/ODE ==
  Room_Volume : Inport
  CO_people : Inport  Port=2
  Air_Intake : Inport  Port=3
  CO2_out : Inport  Port=4
  CO2_init : Constant  Value=430
  Divide : Product  Inputs=*/
  Integrator : Integrator  InitialConditionSource=external
  Product : Product
  Sum : Sum  Inputs=|+-
  Sum1 : Sum
  Out1 : Outport
  Out2 : Outport  Port=2
  wires:
  Air_Intake/1 -> Product/1
  Room_Volume/1 -> Divide/2
  Product/1 -> Sum1/2
  CO2_out/1 -> Sum/1
  Integrator/1 -> Sum/2, Out2/1, Out1/1
  Sum/1 -> Product/2
  CO2_init/1 -> Integrator/2
  CO_people/1 -> Sum1/1
  Divide/1 -> Integrator/1
  Sum1/1 -> Divide/1

== system Wall_Model_Version_Final_2018a/DISPLAY1/ODE1 ==
  Room_Volume : Inport
  Air_Intake : Inport  Port=2
  CO_out : Inport  Port=3
  CO_init : Constant  Value=0
  Divide : Product  Inputs=*/
  Integrator : Integrator  InitialConditionSource=external
  Product : Product
  Sum : Sum  Inputs=|+-
  Out1 : Outport
  Out2 : Outport  Port=2
  wires:
  Air_Intake/1 -> Product/1
  Room_Volume/1 -> Divide/2
  CO_out/1 -> Sum/1
  Sum/1 -> Product/2
  CO_init/1 -> Integrator/2
  Divide/1 -> Integrator/1
  Product/1 -> Divide/1
  Integrator/1 -> Sum/2, Out2/1, Out1/1

== system Wall_Model_Version_Final_2018a/DISPLAY1/ODE2 ==
  Room_Volume : Inport
  Air_Intake : Inport  Port=2
  HCHO_out : Inport  Port=3
  Divide : Product  Inputs=*/
  HCHO_init : Constant  Value=0
  Integrator : Integrator  InitialConditionSource=external
  Product : Product
  Sum : Sum  Inputs=|+-
  Out1 : Outport
  Out2 : Outport  Port=2
  wires:
  Air_Intake/1 -> Product/1
  Room_Volume/1 -> Divide/2
  HCHO_out/1 -> Sum/1
  Integrator/1 -> Sum/2, Out2/1, Out1/1
  Sum/1 -> Product/2
  HCHO_init/1 -> Integrator/2
  Divide/1 -> Integrator/1
  Product/1 -> Divide/1

== system Wall_Model_Version_Final_2018a/DISPLAY1/ODE3 ==
  Room_Volume : Inport
  Air_Intake : Inport  Port=2
  O3_out : Inport  Port=3
  Divide : Product  Inputs=*/
  Integrator : Integrator  InitialConditionSource=external
  O3_init : Constant  Value=0
  Product : Product
  Sum : Sum  Inputs=|+-
  Out1 : Outport
  Out2 : Outport  Port=2
  wires:
  Air_Intake/1 -> Product/1
  Room_Volume/1 -> Divide/2
  O3_out/1 -> Sum/1
  Integrator/1 -> Sum/2, Out2/1, Out1/1
  Sum/1 -> Product/2
  O3_init/1 -> Integrator/2
  Divide/1 -> Integrator/1
  Product/1 -> Divide/1

== system Wall_Model_Version_Final_2018a/DISPLAY1/ODE5 ==
  Room_Volume : Inport
  Air_Intake : Inport  Port=2
  PM2_5_out : Inport  Port=3
  Divide : Product  Inputs=*/
  Integrator : Integrator  InitialConditionSource=external
  PM2_5_init : Constant  Value=0
  Product : Product
  Sum : Sum  Inputs=|+-
  Out1 : Outport
  Out2 : Outport  Port=2
  wires:
  Air_Intake/1 -> Product/1
  Room_Volume/1 -> Divide/2
  PM2_5_out/1 -> Sum/1
  Integrator/1 -> Sum/2, Out2/1, Out1/1
  Sum/1 -> Product/2
  PM2_5_init/1 -> Integrator/2
  Divide/1 -> Integrator/1
  Product/1 -> Divide/1

== system Wall_Model_Version_Final_2018a/DISPLAY1/ODE6 ==
  Room_Volume : Inport
  Air_Intake : Inport  Port=2
  PM10_out : Inport  Port=3
  Divide : Product  Inputs=*/
  Integrator : Integrator  InitialConditionSource=external
  PM10_init : Constant  Value=0
  Product : Product
  Sum : Sum  Inputs=|+-
  Out1 : Outport
  Out2 : Outport  Port=2
  wires:
  Product/1 -> Divide/1
  Divide/1 -> Integrator/1
  PM10_init/1 -> Integrator/2
  Sum/1 -> Product/2
  Integrator/1 -> Out2/1, Out1/1, Sum/2
  PM10_out/1 -> Sum/1
  Room_Volume/1 -> Divide/2
  Air_Intake/1 -> Product/1

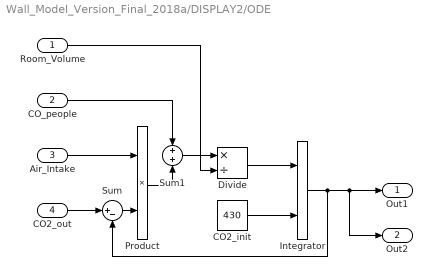
== system Wall_Model_Version_Final_2018a/DISPLAY2/ODE ==
  Room_Volume : Inport
  CO_people : Inport  Port=2
  Air_Intake : Inport  Port=3
  CO2_out : Inport  Port=4
  CO2_init : Constant  Value=430
  Divide : Product  Inputs=*/
  Integrator : Integrator  InitialConditionSource=external
  Product : Product
  Sum : Sum  Inputs=|+-
  Sum1 : Sum
  Out1 : Outport
  Out2 : Outport  Port=2
  wires:
  Air_Intake/1 -> Product/1
  Room_Volume/1 -> Divide/2
  Product/1 -> Sum1/2
  CO2_out/1 -> Sum/1
  Integrator/1 -> Sum/2, Out2/1, Out1/1
  Sum/1 -> Product/2
  CO2_init/1 -> Integrator/2
  CO_people/1 -> Sum1/1
  Divide/1 -> Integrator/1
  Sum1/1 -> Divide/1

== system Wall_Model_Version_Final_2018a/DISPLAY2/ODE1 ==
  Room_Volume : Inport
  Air_Intake : Inport  Port=2
  CO_out : Inport  Port=3
  CO_init : Constant  Value=0
  Divide : Product  Inputs=*/
  Integrator : Integrator  InitialConditionSource=external
  Product : Product
  Sum : Sum  Inputs=|+-
  Out1 : Outport
  Out2 : Outport  Port=2
  wires:
  Air_Intake/1 -> Product/1
  Room_Volume/1 -> Divide/2
  CO_out/1 -> Sum/1
  Sum/1 -> Product/2
  CO_init/1 -> Integrator/2
  Divide/1 -> Integrator/1
  Product/1 -> Divide/1
  Integrator/1 -> Sum/2, Out2/1, Out1/1

== system Wall_Model_Version_Final_2018a/DISPLAY2/ODE2 ==
  Room_Volume : Inport
  Air_Intake : Inport  Port=2
  HCHO_out : Inport  Port=3
  Divide : Product  Inputs=*/
  HCHO_init : Constant  Value=0
  Integrator : Integrator  InitialConditionSource=external
  Product : Product
  Sum : Sum  Inputs=|+-
  Out1 : Outport
  Out2 : Outport  Port=2
  wires:
  Air_Intake/1 -> Product/1
  Room_Volume/1 -> Divide/2
  HCHO_out/1 -> Sum/1
  Integrator/1 -> Sum/2, Out2/1, Out1/1
  Sum/1 -> Product/2
  HCHO_init/1 -> Integrator/2
  Divide/1 -> Integrator/1
  Product/1 -> Divide/1

== system Wall_Model_Version_Final_2018a/DISPLAY2/ODE3 ==
  Room_Volume : Inport
  Air_Intake : Inport  Port=2
  O3_out : Inport  Port=3
  Divide : Product  Inputs=*/
  Integrator : Integrator  InitialConditionSource=external
  O3_init : Constant  Value=0
  Product : Product
  Sum : Sum  Inputs=|+-
  Out1 : Outport
  Out2 : Outport  Port=2
  wires:
  Air_Intake/1 -> Product/1
  Room_Volume/1 -> Divide/2
  O3_out/1 -> Sum/1
  Integrator/1 -> Sum/2, Out2/1, Out1/1
  Sum/1 -> Product/2
  O3_init/1 -> Integrator/2
  Divide/1 -> Integrator/1
  Product/1 -> Divide/1

== system Wall_Model_Version_Final_2018a/DISPLAY2/ODE5 ==
  Room_Volume : Inport
  Air_Intake : Inport  Port=2
  PM2_5_out : Inport  Port=3
  Divide : Product  Inputs=*/
  Integrator : Integrator  InitialConditionSource=external
  PM2_5_init : Constant  Value=0
  Product : Product
  Sum : Sum  Inputs=|+-
  Out1 : Outport
  Out2 : Outport  Port=2
  wires:
  Air_Intake/1 -> Product/1
  Room_Volume/1 -> Divide/2
  PM2_5_out/1 -> Sum/1
  Integrator/1 -> Sum/2, Out2/1, Out1/1
  Sum/1 -> Product/2
  PM2_5_init/1 -> Integrator/2
  Divide/1 -> Integrator/1
  Product/1 -> Divide/1

== system Wall_Model_Version_Final_2018a/DISPLAY2/ODE6 ==
  Room_Volume : Inport
  Air_Intake : Inport  Port=2
  PM10_out : Inport  Port=3
  Divide : Product  Inputs=*/
  Integrator : Integrator  InitialConditionSource=external
  PM10_init : Constant  Value=0
  Product : Product
  Sum : Sum  Inputs=|+-
  Out1 : Outport
  Out2 : Outport  Port=2
  wires:
  Product/1 -> Divide/1
  Divide/1 -> Integrator/1
  PM10_init/1 -> Integrator/2
  Sum/1 -> Product/2
  Integrator/1 -> Out2/1, Out1/1, Sum/2
  PM10_out/1 -> Sum/1
  Room_Volume/1 -> Divide/2
  Air_Intake/1 -> Product/1

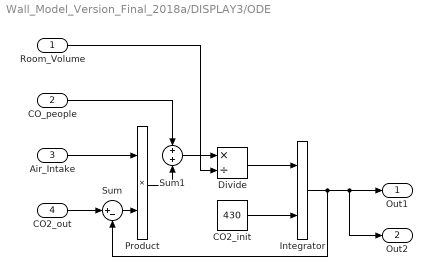
== system Wall_Model_Version_Final_2018a/DISPLAY3/ODE ==
  Room_Volume : Inport
  CO_people : Inport  Port=2
  Air_Intake : Inport  Port=3
  CO2_out : Inport  Port=4
  CO2_init : Constant  Value=430
  Divide : Product  Inputs=*/
  Integrator : Integrator  InitialConditionSource=external
  Product : Product
  Sum : Sum  Inputs=|+-
  Sum1 : Sum
  Out1 : Outport
  Out2 : Outport  Port=2
  wires:
  Air_Intake/1 -> Product/1
  Room_Volume/1 -> Divide/2
  Product/1 -> Sum1/2
  CO2_out/1 -> Sum/1
  Integrator/1 -> Sum/2, Out2/1, Out1/1
  Sum/1 -> Product/2
  CO2_init/1 -> Integrator/2
  CO_people/1 -> Sum1/1
  Divide/1 -> Integrator/1
  Sum1/1 -> Divide/1

== system Wall_Model_Version_Final_2018a/DISPLAY3/ODE1 ==
  Room_Volume : Inport
  Air_Intake : Inport  Port=2
  CO_out : Inport  Port=3
  CO_init : Constant  Value=0
  Divide : Product  Inputs=*/
  Integrator : Integrator  InitialConditionSource=external
  Product : Product
  Sum : Sum  Inputs=|+-
  Out1 : Outport
  Out2 : Outport  Port=2
  wires:
  Air_Intake/1 -> Product/1
  Room_Volume/1 -> Divide/2
  CO_out/1 -> Sum/1
  Sum/1 -> Product/2
  CO_init/1 -> Integrator/2
  Divide/1 -> Integrator/1
  Product/1 -> Divide/1
  Integrator/1 -> Sum/2, Out2/1, Out1/1

== system Wall_Model_Version_Final_2018a/DISPLAY3/ODE2 ==
  Room_Volume : Inport
  Air_Intake : Inport  Port=2
  HCHO_out : Inport  Port=3
  Divide : Product  Inputs=*/
  HCHO_init : Constant  Value=0
  Integrator : Integrator  InitialConditionSource=external
  Product : Product
  Sum : Sum  Inputs=|+-
  Out1 : Outport
  Out2 : Outport  Port=2
  wires:
  Air_Intake/1 -> Product/1
  Room_Volume/1 -> Divide/2
  HCHO_out/1 -> Sum/1
  Integrator/1 -> Sum/2, Out2/1, Out1/1
  Sum/1 -> Product/2
  HCHO_init/1 -> Integrator/2
  Divide/1 -> Integrator/1
  Product/1 -> Divide/1

== system Wall_Model_Version_Final_2018a/DISPLAY3/ODE3 ==
  Room_Volume : Inport
  Air_Intake : Inport  Port=2
  O3_out : Inport  Port=3
  Divide : Product  Inputs=*/
  Integrator : Integrator  InitialConditionSource=external
  O3_init : Constant  Value=0
  Product : Product
  Sum : Sum  Inputs=|+-
  Out1 : Outport
  Out2 : Outport  Port=2
  wires:
  Air_Intake/1 -> Product/1
  Room_Volume/1 -> Divide/2
  O3_out/1 -> Sum/1
  Integrator/1 -> Sum/2, Out2/1, Out1/1
  Sum/1 -> Product/2
  O3_init/1 -> Integrator/2
  Divide/1 -> Integrator/1
  Product/1 -> Divide/1

== system Wall_Model_Version_Final_2018a/DISPLAY3/ODE5 ==
  Room_Volume : Inport
  Air_Intake : Inport  Port=2
  PM2_5_out : Inport  Port=3
  Divide : Product  Inputs=*/
  Integrator : Integrator  InitialConditionSource=external
  PM2_5_init : Constant  Value=0
  Product : Product
  Sum : Sum  Inputs=|+-
  Out1 : Outport
  Out2 : Outport  Port=2
  wires:
  Air_Intake/1 -> Product/1
  Room_Volume/1 -> Divide/2
  PM2_5_out/1 -> Sum/1
  Integrator/1 -> Sum/2, Out2/1, Out1/1
  Sum/1 -> Product/2
  PM2_5_init/1 -> Integrator/2
  Divide/1 -> Integrator/1
  Product/1 -> Divide/1

== system Wall_Model_Version_Final_2018a/DISPLAY3/ODE6 ==
  Room_Volume : Inport
  Air_Intake : Inport  Port=2
  PM10_out : Inport  Port=3
  Divide : Product  Inputs=*/
  Integrator : Integrator  InitialConditionSource=external
  PM10_init : Constant  Value=0
  Product : Product
  Sum : Sum  Inputs=|+-
  Out1 : Outport
  Out2 : Outport  Port=2
  wires:
  Product/1 -> Divide/1
  Divide/1 -> Integrator/1
  PM10_init/1 -> Integrator/2
  Sum/1 -> Product/2
  Integrator/1 -> Out2/1, Out1/1, Sum/2
  PM10_out/1 -> Sum/1
  Room_Volume/1 -> Divide/2
  Air_Intake/1 -> Product/1

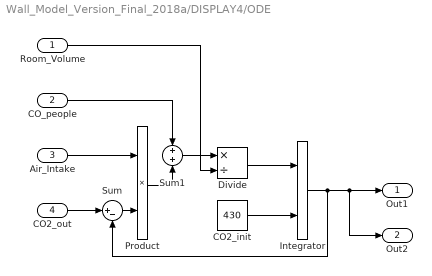
== system Wall_Model_Version_Final_2018a/DISPLAY4/ODE ==
  Room_Volume : Inport
  CO_people : Inport  Port=2
  Air_Intake : Inport  Port=3
  CO2_out : Inport  Port=4
  CO2_init : Constant  Value=430
  Divide : Product  Inputs=*/
  Integrator : Integrator  InitialConditionSource=external
  Product : Product
  Sum : Sum  Inputs=|+-
  Sum1 : Sum
  Out1 : Outport
  Out2 : Outport  Port=2
  wires:
  Air_Intake/1 -> Product/1
  Room_Volume/1 -> Divide/2
  Product/1 -> Sum1/2
  CO2_out/1 -> Sum/1
  Integrator/1 -> Sum/2, Out2/1, Out1/1
  Sum/1 -> Product/2
  CO2_init/1 -> Integrator/2
  CO_people/1 -> Sum1/1
  Divide/1 -> Integrator/1
  Sum1/1 -> Divide/1

== system Wall_Model_Version_Final_2018a/DISPLAY4/ODE1 ==
  Room_Volume : Inport
  Air_Intake : Inport  Port=2
  CO_out : Inport  Port=3
  CO_init : Constant  Value=0
  Divide : Product  Inputs=*/
  Integrator : Integrator  InitialConditionSource=external
  Product : Product
  Sum : Sum  Inputs=|+-
  Out1 : Outport
  Out2 : Outport  Port=2
  wires:
  Air_Intake/1 -> Product/1
  Room_Volume/1 -> Divide/2
  CO_out/1 -> Sum/1
  Sum/1 -> Product/2
  CO_init/1 -> Integrator/2
  Divide/1 -> Integrator/1
  Product/1 -> Divide/1
  Integrator/1 -> Sum/2, Out2/1, Out1/1

== system Wall_Model_Version_Final_2018a/DISPLAY4/ODE2 ==
  Room_Volume : Inport
  Air_Intake : Inport  Port=2
  HCHO_out : Inport  Port=3
  Divide : Product  Inputs=*/
  HCHO_init : Constant  Value=0
  Integrator : Integrator  InitialConditionSource=external
  Product : Product
  Sum : Sum  Inputs=|+-
  Out1 : Outport
  Out2 : Outport  Port=2
  wires:
  Air_Intake/1 -> Product/1
  Room_Volume/1 -> Divide/2
  HCHO_out/1 -> Sum/1
  Integrator/1 -> Sum/2, Out2/1, Out1/1
  Sum/1 -> Product/2
  HCHO_init/1 -> Integrator/2
  Divide/1 -> Integrator/1
  Product/1 -> Divide/1

== system Wall_Model_Version_Final_2018a/DISPLAY4/ODE3 ==
  Room_Volume : Inport
  Air_Intake : Inport  Port=2
  O3_out : Inport  Port=3
  Divide : Product  Inputs=*/
  Integrator : Integrator  InitialConditionSource=external
  O3_init : Constant  Value=0
  Product : Product
  Sum : Sum  Inputs=|+-
  Out1 : Outport
  Out2 : Outport  Port=2
  wires:
  Air_Intake/1 -> Product/1
  Room_Volume/1 -> Divide/2
  O3_out/1 -> Sum/1
  Integrator/1 -> Sum/2, Out2/1, Out1/1
  Sum/1 -> Product/2
  O3_init/1 -> Integrator/2
  Divide/1 -> Integrator/1
  Product/1 -> Divide/1

== system Wall_Model_Version_Final_2018a/DISPLAY4/ODE5 ==
  Room_Volume : Inport
  Air_Intake : Inport  Port=2
  PM2_5_out : Inport  Port=3
  Divide : Product  Inputs=*/
  Integrator : Integrator  InitialConditionSource=external
  PM2_5_init : Constant  Value=0
  Product : Product
  Sum : Sum  Inputs=|+-
  Out1 : Outport
  Out2 : Outport  Port=2
  wires:
  Air_Intake/1 -> Product/1
  Room_Volume/1 -> Divide/2
  PM2_5_out/1 -> Sum/1
  Integrator/1 -> Sum/2, Out2/1, Out1/1
  Sum/1 -> Product/2
  PM2_5_init/1 -> Integrator/2
  Divide/1 -> Integrator/1
  Product/1 -> Divide/1

== system Wall_Model_Version_Final_2018a/DISPLAY4/ODE6 ==
  Room_Volume : Inport
  Air_Intake : Inport  Port=2
  PM10_out : Inport  Port=3
  Divide : Product  Inputs=*/
  Integrator : Integrator  InitialConditionSource=external
  PM10_init : Constant  Value=0
  Product : Product
  Sum : Sum  Inputs=|+-
  Out1 : Outport
  Out2 : Outport  Port=2
  wires:
  Product/1 -> Divide/1
  Divide/1 -> Integrator/1
  PM10_init/1 -> Integrator/2
  Sum/1 -> Product/2
  Integrator/1 -> Out2/1, Out1/1, Sum/2
  PM10_out/1 -> Sum/1
  Room_Volume/1 -> Divide/2
  Air_Intake/1 -> Product/1

== system Wall_Model_Version_Final_2018a/ROOM/Back_Wall ==
  note: T1
  note: Back Wall
  In1 : Inport
  Disp_Function : M-S-Function  FunctionName=fn_Display_wall
  Ground1 : powerlib/Elements/Ground  LConnTagsString=a
      settings: SourceProductName=Simscape Electrical
  Ground2 : powerlib/Elements/Ground  LConnTagsString=a
      settings: SourceProductName=Simscape Electrical
  Ground3 : powerlib/Elements/Ground  LConnTagsString=a
      settings: SourceProductName=Simscape Electrical
  V : powerlib/Electrical Sources/Controlled Voltage Source  Initialize=on  Source_Type=AC  Amplitude=0  Phase=0  Frequency=0  Measurements=None
      settings: SourceProductName=Simscape Electrical
  x10*Rth4 : powerlib/Elements/Series RLC Branch  LConnTagsString=__new0  RConnTagsString=__new0  BranchType=R  Resistance=x10*Rth4  Inductance=1e-3  SetiL0=off  InitialCurrent=0  Capacitance=1e-6  Setx0=off  InitialVoltage=0  Measurements=None
      settings: SourceProductName=Simscape Electrical
  x11*Rth4 : powerlib/Elements/Series RLC Branch  LConnTagsString=__new0  RConnTagsString=__new0  BranchType=R  Resistance=x11*Rth4  Inductance=1e-3  SetiL0=off  InitialCurrent=0  Capacitance=1e-6  Setx0=off  InitialVoltage=0  Measurements=None
      settings: SourceProductName=Simscape Electrical
  y7*Cth4 : powerlib/Elements/Series RLC Branch  LConnTagsString=__new0  RConnTagsString=__new0  BranchType=C  Resistance=0  Inductance=1e-3  SetiL0=off  InitialCurrent=0  Capacitance=y7*Cth4  Setx0=on  InitialVoltage=T1_initial_back  Measurements=Branch voltage
      settings: SourceProductName=Simscape Electrical
  Conn1 : PMIOPort  Side=Right
  wires:
  In1/1 -> Disp_Function/1, V/1
  connections:
  Ground2/LConn1 -- V/LConn1
  V/RConn1 -- x10*Rth4/LConn1
  x10*Rth4/RConn1 -- x11*Rth4/LConn1
  Ground1/LConn1 -- y7*Cth4/RConn1
  x11*Rth4/RConn1 -- Conn1/RConn1
  Ground3/LConn1 -- y7*Cth4/LConn1

== system Wall_Model_Version_Final_2018a/ROOM/Equipment Heat ==
  In1 : Inport
  Ground20 : powerlib/Elements/Ground  LConnTagsString=a
      settings: SourceProductName=Simscape Electrical
  I1 : powerlib/Electrical Sources/Controlled Current Source  Initialize=off  Source_Type=AC  Amplitude=1  Phase=0  Frequency=0  Measurements=None
      settings: SourceProductName=Simscape Electrical
  Conn1 : PMIOPort  Side=Right
  wires:
  In1/1 -> I1/1
  connections:
  Ground20/LConn1 -- I1/LConn1
  I1/RConn1 -- Conn1/RConn1
